simulink model "decoupling_hamna"  (R2025b)
settings: Solver=VariableStepAuto  StartTime=0.0  StopTime=10.0  RelTol=1e-3
settings Model: Creator=3 Stars Laptop  LastModifiedBy=3 Stars Laptop

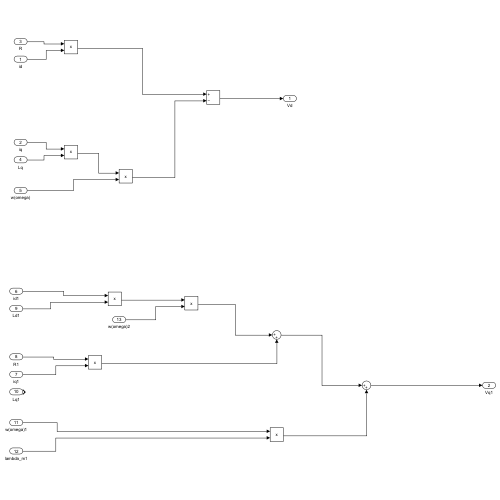
[thumbnail: Simulink's stored preview of the top-level diagram]
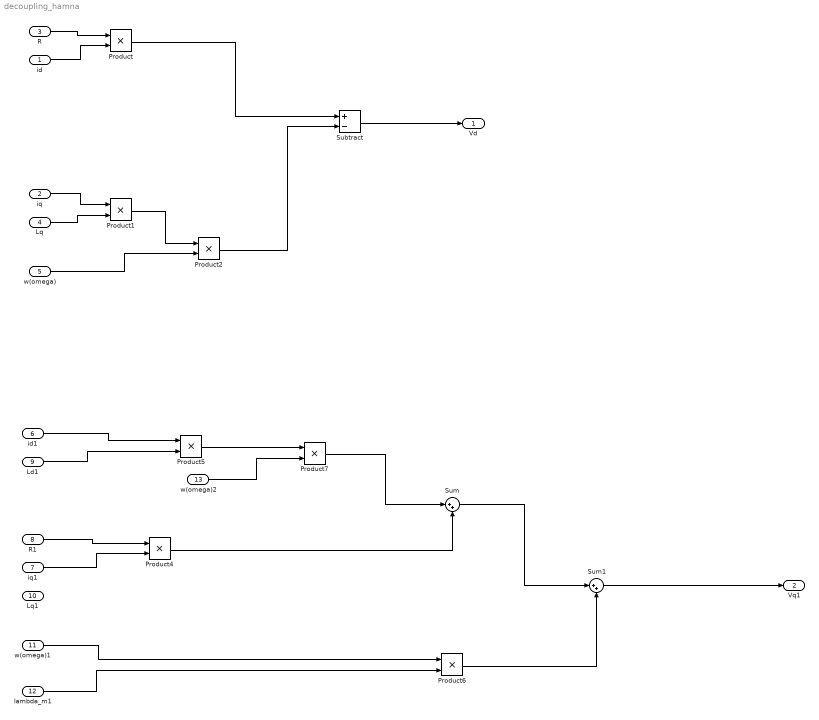
== system decoupling_hamna ==
  id : Inport
  iq : Inport  Port=2
  R : Inport  Port=3
  Lq : Inport  Port=4
  w(omega) : Inport  Port=5
  id1 : Inport  Port=6
  iq1 : Inport  Port=7
  R1 : Inport  Port=8
  Ld1 : Inport  Port=9
  Lq1 : Inport  Port=10
  w(omega)1 : Inport  Port=11
  lambda_m1 : Inport  Port=12
  w(omega)2 : Inport  Port=13
  Product{,1..2,4..7} (7 alike) : Product
  Subtract : Sum  Inputs=+-
  Sum : Sum  Inputs=|++
  Sum1 : Sum  Inputs=|++
  Vd : Outport
  Vq1 : Outport  Port=2
  wires:
  R/1 -> Product/1
  id/1 -> Product/2
  iq/1 -> Product1/1
  Lq/1 -> Product1/2
  Product1/1 -> Product2/1
  w(omega)/1 -> Product2/2
  Product/1 -> Subtract/1
  Product2/1 -> Subtract/2
  Subtract/1 -> Vd/1
  R1/1 -> Product4/1
  iq1/1 -> Product4/2
  id1/1 -> Product5/1
  Ld1/1 -> Product5/2
  w(omega)1/1 -> Product6/1
  lambda_m1/1 -> Product6/2
  Product5/1 -> Product7/1
  w(omega)2/1 -> Product7/2
  Product7/1 -> Sum/1
  Product4/1 -> Sum/2
  Sum/1 -> Sum1/1
  Product6/1 -> Sum1/2
  Sum1/1 -> Vq1/1
